simulink model "lab4_2"  (R2020a)
settings: Solver=VariableStepAuto  StartTime=0.0  StopTime=10.0  RelTol=1e-3
values from neighbouring files (symbols this model uses):
  d_bar = (Ra/Kt)*tau_l    (= 3)    [lab4.m]
  thetades = pi / 2    (= 1.57079632679)    [lab4.m]
  TI = 10 / omega_c    [lab4.m]
  Vlim = 5    [lab4.m]
undefined symbols (not defined in the file or in its folder): Kaw
libraries: cstblocks x2
settings Model: Creator=zhoutanq  LastModifiedBy=spencersun
settings DebuggingCC: SFMachineParentedDataDiag=error

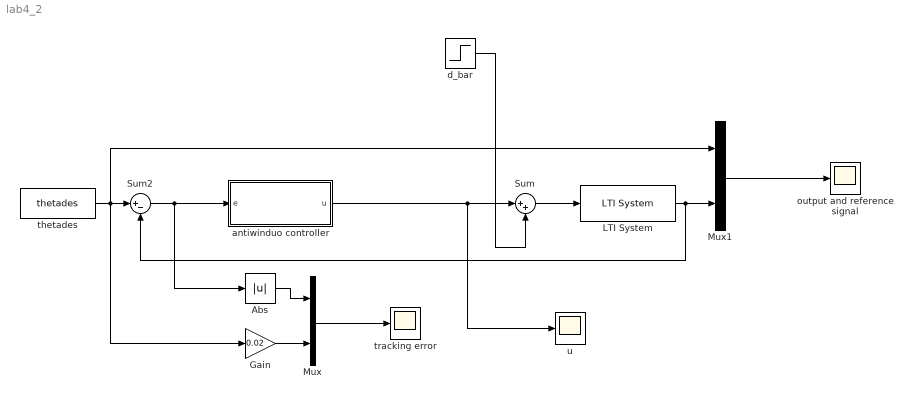
== system lab4_2 ==
  Abs : Abs
  Gain : Gain  Gain=0.02
  LTI System : cstblocks/LTI System  sys=G  IC=[]
  Mux : Mux  Inputs=2
  Mux1 : Mux  Inputs=2
  Sum : Sum  Inputs=|++
  Sum2 : Sum  Inputs=|+-
  antiwinduo controller : Subsystem
  d_bar : Step  Time=5  After=d_bar  SampleTime=0
  output and reference signal : Scope
  thetades : Constant  Value=thetades
  tracking error : Scope
  u : Scope
  wires:
  Mux/1 -> tracking error/1
  Abs/1 -> Mux/1
  antiwinduo controller/1(u) -> u/1, Sum/1
  Gain/1 -> Mux/2
  d_bar/1 -> Sum/2
  LTI System/1 -> Sum2/2, Mux1/2
  Sum2/1 -> antiwinduo controller/1(e), Abs/1
  Sum/1 -> LTI System/1
  Mux1/1 -> output and reference signal/1
  thetades/1 -> Mux1/1, Gain/1, Sum2/1

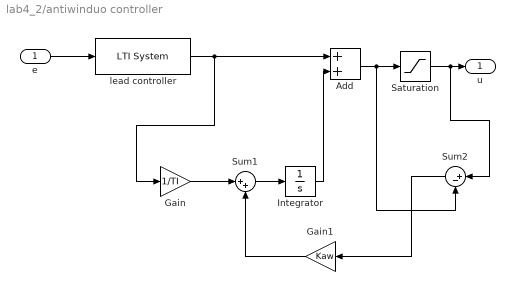
== system lab4_2/antiwinduo controller ==
  e : Inport
  Add : Sum
  Gain : Gain  Gain=1/TI
  Gain1 : Gain  Gain=Kaw
  Integrator : Integrator
  Saturation : Saturate  UpperLimit=Vlim  LowerLimit=-Vlim
  Sum1 : Sum  Inputs=|++
  Sum2 : Sum  Inputs=|+-
  lead controller : cstblocks/LTI System  sys=C1  IC=[]
  u : Outport
  wires:
  e/1 -> lead controller/1
  Saturation/1 -> Sum2/1, u/1
  Add/1 -> Sum2/2, Saturation/1
  lead controller/1 -> Gain/1, Add/1
  Gain/1 -> Sum1/1
  Sum2/1 -> Gain1/1
  Gain1/1 -> Sum1/2
  Integrator/1 -> Add/2
  Sum1/1 -> Integrator/1
